simulink model "untitled1"  (R2014b)
settings: Solver=ode45  StartTime=0.0  StopTime=10.0  RelTol=1e-3
settings Model: Creator=rajab  LastModifiedBy=rajab

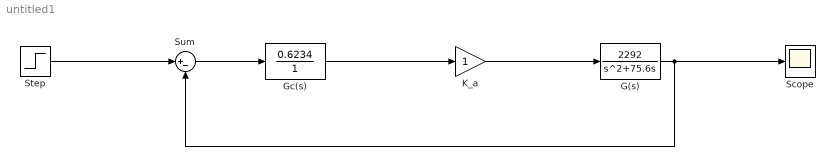
== system untitled1 ==
  G(s) : TransferFcn  Numerator=[2292]  Denominator=[1 75.6 0]
  Gc(s) : TransferFcn  Numerator=[0.6234]  Denominator=1
  K_a : Gain
  Scope : Scope
  Step : Step  SampleTime=0
  Sum : Sum  Inputs=|+-
  wires:
  Gc(s)/1 -> K_a/1
  K_a/1 -> G(s)/1
  G(s)/1 -> Scope/1, Sum/2
  Sum/1 -> Gc(s)/1
  Step/1 -> Sum/1
